simulink model "experiment_toplevel"  (R2016a)
settings: Solver=ode15s  StartTime=0.0  StopTime=20  MaxStep=1e-2  RelTol=1e-4
PreLoadFcn:
  | minitaurParameters
values from neighbouring files (symbols this model uses):
  angular_ctrl_d = 1    [minitaurParameters.m]
  angular_ctrl_i = 1    [minitaurParameters.m]
  angular_ctrl_p = 100    [minitaurParameters.m]
  enc_zero_IA = -1.25*pi    (= -3.92699081699)    [minitaurParameters.m]
  enc_zero_IB = -0.25*pi    (= -0.785398163397)    [minitaurParameters.m]
  enc_zero_IIA = 1.25*pi    (= 3.92699081699)    [minitaurParameters.m]
  enc_zero_IIB = 1.25*pi    (= 3.92699081699)    [minitaurParameters.m]
  enc_zero_IIIA = 0.5*pi    (= 1.57079632679)    [minitaurParameters.m]
  enc_zero_IIIB = 1.5*pi    (= 4.71238898038)    [minitaurParameters.m]
  enc_zero_IVA = -0.25*pi    (= -0.785398163397)    [minitaurParameters.m]
  enc_zero_IVB = 0.5*pi    (= 1.57079632679)    [minitaurParameters.m]
  fore_lag = fore_lag_vals(j)    [experiment1.m]    (also in experiment1_parfor_accelerator.m = 0; minitaurParameters.m = 0.45)
  ground_frame_depth = 0.5    [minitaurParameters.m]
  ground_length = 100    [minitaurParameters.m]
  ground_width = 10    [minitaurParameters.m]
  init_theta_IA = -pi/4    (= -0.785398163397)    [minitaurParameters.m]
  init_theta_IB = pi/4    (= 0.785398163397)    [minitaurParameters.m]
  init_theta_IIA = -pi/4    (= -0.785398163397)    [minitaurParameters.m]
  init_theta_IIB = pi/4    (= 0.785398163397)    [minitaurParameters.m]
  init_theta_IIIA = -pi/4    (= -0.785398163397)    [minitaurParameters.m]
  init_theta_IIIB = pi/4    (= 0.785398163397)    [minitaurParameters.m]
  init_theta_IVA = -pi/4    (= -0.785398163397)    [minitaurParameters.m]
  init_theta_IVB = pi/4    (= 0.785398163397)    [minitaurParameters.m]
  l1 = 100e-3    (= 0.1)    [minitaurParameters.m]
  l2 = 200e-3    (= 0.2)    [minitaurParameters.m]
  leg_joint_radius = 3e-3    (= 0.003)    [minitaurParameters.m]
  lr_sync = 1    [experiment1.m]    (also in experiment1_parfor_accelerator.m; minitaurParameters.m = 0)
  model = 'experiment_toplevel'    [experiment1_parfor_accelerator.m]
  period = period_vals(i)    [experiment1.m]    (also in experiment1_parfor_accelerator.m = 1.5; minitaurParameters.m = 0.33)
  phi_0 = 0.5*asin(l1/l2)    [experiment1.m]    (also in experiment1_parfor_accelerator.m; minitaurParameters.m)
  r_0 = l2    [experiment1.m]    (also in experiment1_parfor_accelerator.m; minitaurParameters.m = 0.2)
  r_x = 0.3*l1    [experiment1.m]    (also in experiment1_parfor_accelerator.m = 0.5*l1; minitaurParameters.m = 0.05)
  r_y = 0.2*l1    [experiment1.m]    (also in experiment1_parfor_accelerator.m = 0.3*l1; minitaurParameters.m = 0.03)
  radial_ctrl_d = 1    [minitaurParameters.m]
  radial_ctrl_i = 1    [minitaurParameters.m]
  radial_ctrl_p = 80    [minitaurParameters.m]
  safety_limit = 10e-3    (= 0.01)    [minitaurParameters.m]
undefined symbols (not defined in the file or in its folder): Axis, Fn, minitaurParams, r_stance, r_swing, stance_frac, X, Y, Z
undefined symbols (not defined in the file): leg_joint_fric_bw, leg_joint_mu_k, leg_joint_mu_s, leg_joint_vel_thresh, motor_kt, motor_kv, motor_r, motor_torque_sat
libraries: sm_lib x453, fl_lib x132, nesl_utility x31, Contact_Forces_Lib x28, simulink x19
(part 11 of 13)

== system experiment_toplevel/GR Minitaur/minitaur_leg_linkages_I/Joint Friction Model/Full ==
  Ideal Force Sensor : fl_lib/Mechanical/Mechanical Sensors/Ideal Force Sensor
  Ideal Translational Velocity Source : fl_lib/Mechanical/Mechanical Sources/Ideal Translational Velocity Source
  Joint Diameter : fl_lib/Physical Signals/Functions/PS Gain  gain=2*leg_joint_radius
  Joint Radius : fl_lib/Physical Signals/Functions/PS Gain  gain=leg_joint_radius
  Mechanical Translational Reference : fl_lib/Mechanical/Translational Elements/Mechanical Translational Reference
  Mechanical Translational Reference1 : fl_lib/Mechanical/Translational Elements/Mechanical Translational Reference
  PS Terminator : fl_lib/Physical Signals/Sinks/PS Terminator
  Translational Friction : fl_lib/Mechanical/Translational Elements/Translational Friction  brkwy_frc=mu_brk*Fn N  Col_frc=mu_k*Fn N  visc_coef=fric_visc_coeff N/(m/s)  trans_coef=trans_coeff s/m  vel_thr=linear_region_thresh m/s  v_specify=off  v_priority=None  v=0 m/s  f_specify=off  f_priority=None  f=0 N
  Joint Angular Velocity : PMIOPort  Port=1  Side=Left
  Joint Force : PMIOPort  Port=2  Side=Left
  Friction Torque : PMIOPort  Port=3  Side=Right
  connections:
  Mechanical Translational Reference/LConn1 -- Ideal Force Sensor/RConn1
  Translational Friction/LConn1 -- Ideal Force Sensor/LConn1
  Translational Friction/RConn1 -- Ideal Translational Velocity Source/LConn1
  Ideal Force Sensor/RConn2 -- Joint Diameter/LConn1
  Joint Diameter/RConn1 -- Friction Torque/RConn1
  Mechanical Translational Reference1/LConn1 -- Ideal Translational Velocity Source/RConn2
  Joint Force/RConn1 -- PS Terminator/LConn1
  Joint Radius/LConn1 -- Joint Angular Velocity/RConn1
  Joint Radius/RConn1 -- Ideal Translational Velocity Source/RConn1

== system experiment_toplevel/GR Minitaur/minitaur_leg_linkages_I/Joint Friction Model/Stick-Slip ==
  Joint Diameter : fl_lib/Physical Signals/Functions/PS Gain  gain=2*leg_joint_radius
  Joint Radius : fl_lib/Physical Signals/Functions/PS Gain  gain=leg_joint_radius
  PS Add : fl_lib/Physical Signals/Functions/PS Add
  Stick-Slip Friction X : Contact_Forces_Lib/Friction Utilities/Stick-Slip Friction 1D  fn_axis=X-Axis  mu_kinetic=mu_k/2  mu_static=mu_s/2  vel_th=linear_region_thresh  filt_const=1/(2*pi*fric_bandwidth)
  Stick-Slip Friction Y : Contact_Forces_Lib/Friction Utilities/Stick-Slip Friction 1D  fn_axis=Y-Axis  mu_kinetic=mu_k/2  mu_static=mu_s/2  vel_th=linear_region_thresh  filt_const=1/(2*pi*fric_bandwidth)
  Joint Angular Velocity : PMIOPort  Port=1  Side=Left
  Joint Force : PMIOPort  Port=2  Side=Left
  Friction Torque : PMIOPort  Port=3  Side=Right
  connections:
  Stick-Slip Friction X/LConn2 -- Stick-Slip Friction Y/LConn2 -- Joint Radius/RConn1
  Joint Force/RConn1 -- Stick-Slip Friction Y/LConn1 -- Stick-Slip Friction X/LConn1
  Stick-Slip Friction Y/RConn1 -- PS Add/LConn2
  Stick-Slip Friction X/RConn1 -- PS Add/LConn1
  Joint Diameter/LConn1 -- PS Add/RConn1
  Joint Diameter/RConn1 -- Friction Torque/RConn1
  Joint Radius/LConn1 -- Joint Angular Velocity/RConn1

== system experiment_toplevel/GR Minitaur/minitaur_leg_linkages_I/Joint Friction Model1/Full ==
  Ideal Force Sensor : fl_lib/Mechanical/Mechanical Sensors/Ideal Force Sensor
  Ideal Translational Velocity Source : fl_lib/Mechanical/Mechanical Sources/Ideal Translational Velocity Source
  Joint Diameter : fl_lib/Physical Signals/Functions/PS Gain  gain=2*leg_joint_radius
  Joint Radius : fl_lib/Physical Signals/Functions/PS Gain  gain=leg_joint_radius
  Mechanical Translational Reference : fl_lib/Mechanical/Translational Elements/Mechanical Translational Reference
  Mechanical Translational Reference1 : fl_lib/Mechanical/Translational Elements/Mechanical Translational Reference
  PS Terminator : fl_lib/Physical Signals/Sinks/PS Terminator
  Translational Friction : fl_lib/Mechanical/Translational Elements/Translational Friction  brkwy_frc=mu_brk*Fn N  Col_frc=mu_k*Fn N  visc_coef=fric_visc_coeff N/(m/s)  trans_coef=trans_coeff s/m  vel_thr=linear_region_thresh m/s  v_specify=off  v_priority=None  v=0 m/s  f_specify=off  f_priority=None  f=0 N
  Joint Angular Velocity : PMIOPort  Port=1  Side=Left
  Joint Force : PMIOPort  Port=2  Side=Left
  Friction Torque : PMIOPort  Port=3  Side=Right
  connections:
  Mechanical Translational Reference/LConn1 -- Ideal Force Sensor/RConn1
  Translational Friction/LConn1 -- Ideal Force Sensor/LConn1
  Translational Friction/RConn1 -- Ideal Translational Velocity Source/LConn1
  Ideal Force Sensor/RConn2 -- Joint Diameter/LConn1
  Joint Diameter/RConn1 -- Friction Torque/RConn1
  Mechanical Translational Reference1/LConn1 -- Ideal Translational Velocity Source/RConn2
  Joint Force/RConn1 -- PS Terminator/LConn1
  Joint Radius/LConn1 -- Joint Angular Velocity/RConn1
  Joint Radius/RConn1 -- Ideal Translational Velocity Source/RConn1

== system experiment_toplevel/GR Minitaur/minitaur_leg_linkages_I/Joint Friction Model1/Stick-Slip ==
  Joint Diameter : fl_lib/Physical Signals/Functions/PS Gain  gain=2*leg_joint_radius
  Joint Radius : fl_lib/Physical Signals/Functions/PS Gain  gain=leg_joint_radius
  PS Add : fl_lib/Physical Signals/Functions/PS Add
  Stick-Slip Friction X : Contact_Forces_Lib/Friction Utilities/Stick-Slip Friction 1D  fn_axis=X-Axis  mu_kinetic=mu_k/2  mu_static=mu_s/2  vel_th=linear_region_thresh  filt_const=1/(2*pi*fric_bandwidth)
  Stick-Slip Friction Y : Contact_Forces_Lib/Friction Utilities/Stick-Slip Friction 1D  fn_axis=Y-Axis  mu_kinetic=mu_k/2  mu_static=mu_s/2  vel_th=linear_region_thresh  filt_const=1/(2*pi*fric_bandwidth)
  Joint Angular Velocity : PMIOPort  Port=1  Side=Left
  Joint Force : PMIOPort  Port=2  Side=Left
  Friction Torque : PMIOPort  Port=3  Side=Right
  connections:
  Joint Radius/RConn1 -- Stick-Slip Friction X/LConn2 -- Stick-Slip Friction Y/LConn2
  Joint Force/RConn1 -- Stick-Slip Friction X/LConn1 -- Stick-Slip Friction Y/LConn1
  Stick-Slip Friction Y/RConn1 -- PS Add/LConn2
  Stick-Slip Friction X/RConn1 -- PS Add/LConn1
  Joint Diameter/LConn1 -- PS Add/RConn1
  Joint Diameter/RConn1 -- Friction Torque/RConn1
  Joint Radius/LConn1 -- Joint Angular Velocity/RConn1

== system experiment_toplevel/GR Minitaur/minitaur_leg_linkages_I/Joint Friction Model2/Full ==
  Ideal Force Sensor : fl_lib/Mechanical/Mechanical Sensors/Ideal Force Sensor
  Ideal Translational Velocity Source : fl_lib/Mechanical/Mechanical Sources/Ideal Translational Velocity Source
  Joint Diameter : fl_lib/Physical Signals/Functions/PS Gain  gain=2*leg_joint_radius
  Joint Radius : fl_lib/Physical Signals/Functions/PS Gain  gain=leg_joint_radius
  Mechanical Translational Reference : fl_lib/Mechanical/Translational Elements/Mechanical Translational Reference
  Mechanical Translational Reference1 : fl_lib/Mechanical/Translational Elements/Mechanical Translational Reference
  PS Terminator : fl_lib/Physical Signals/Sinks/PS Terminator
  Translational Friction : fl_lib/Mechanical/Translational Elements/Translational Friction  brkwy_frc=mu_brk*Fn N  Col_frc=mu_k*Fn N  visc_coef=fric_visc_coeff N/(m/s)  trans_coef=trans_coeff s/m  vel_thr=linear_region_thresh m/s  v_specify=off  v_priority=None  v=0 m/s  f_specify=off  f_priority=None  f=0 N
  Joint Angular Velocity : PMIOPort  Port=1  Side=Left
  Joint Force : PMIOPort  Port=2  Side=Left
  Friction Torque : PMIOPort  Port=3  Side=Right
  connections:
  Mechanical Translational Reference/LConn1 -- Ideal Force Sensor/RConn1
  Translational Friction/LConn1 -- Ideal Force Sensor/LConn1
  Translational Friction/RConn1 -- Ideal Translational Velocity Source/LConn1
  Ideal Force Sensor/RConn2 -- Joint Diameter/LConn1
  Joint Diameter/RConn1 -- Friction Torque/RConn1
  Mechanical Translational Reference1/LConn1 -- Ideal Translational Velocity Source/RConn2
  Joint Force/RConn1 -- PS Terminator/LConn1
  Joint Radius/LConn1 -- Joint Angular Velocity/RConn1
  Joint Radius/RConn1 -- Ideal Translational Velocity Source/RConn1

== system experiment_toplevel/GR Minitaur/minitaur_leg_linkages_I/Joint Friction Model2/Stick-Slip ==
  Joint Diameter : fl_lib/Physical Signals/Functions/PS Gain  gain=2*leg_joint_radius
  Joint Radius : fl_lib/Physical Signals/Functions/PS Gain  gain=leg_joint_radius
  PS Add : fl_lib/Physical Signals/Functions/PS Add
  Stick-Slip Friction X : Contact_Forces_Lib/Friction Utilities/Stick-Slip Friction 1D  fn_axis=X-Axis  mu_kinetic=mu_k/2  mu_static=mu_s/2  vel_th=linear_region_thresh  filt_const=1/(2*pi*fric_bandwidth)
  Stick-Slip Friction Y : Contact_Forces_Lib/Friction Utilities/Stick-Slip Friction 1D  fn_axis=Y-Axis  mu_kinetic=mu_k/2  mu_static=mu_s/2  vel_th=linear_region_thresh  filt_const=1/(2*pi*fric_bandwidth)
  Joint Angular Velocity : PMIOPort  Port=1  Side=Left
  Joint Force : PMIOPort  Port=2  Side=Left
  Friction Torque : PMIOPort  Port=3  Side=Right
  connections:
  Joint Radius/RConn1 -- Stick-Slip Friction X/LConn2 -- Stick-Slip Friction Y/LConn2
  Joint Force/RConn1 -- Stick-Slip Friction X/LConn1 -- Stick-Slip Friction Y/LConn1
  Stick-Slip Friction Y/RConn1 -- PS Add/LConn2
  Stick-Slip Friction X/RConn1 -- PS Add/LConn1
  Joint Diameter/LConn1 -- PS Add/RConn1
  Joint Diameter/RConn1 -- Friction Torque/RConn1
  Joint Radius/LConn1 -- Joint Angular Velocity/RConn1

== system experiment_toplevel/GR Minitaur/minitaur_leg_linkages_II/Joint Friction Model/Full ==
  Ideal Force Sensor : fl_lib/Mechanical/Mechanical Sensors/Ideal Force Sensor
  Ideal Translational Velocity Source : fl_lib/Mechanical/Mechanical Sources/Ideal Translational Velocity Source
  Joint Diameter : fl_lib/Physical Signals/Functions/PS Gain  gain=2*leg_joint_radius
  Joint Radius : fl_lib/Physical Signals/Functions/PS Gain  gain=leg_joint_radius
  Mechanical Translational Reference : fl_lib/Mechanical/Translational Elements/Mechanical Translational Reference
  Mechanical Translational Reference1 : fl_lib/Mechanical/Translational Elements/Mechanical Translational Reference
  PS Terminator : fl_lib/Physical Signals/Sinks/PS Terminator
  Translational Friction : fl_lib/Mechanical/Translational Elements/Translational Friction  brkwy_frc=mu_brk*Fn N  Col_frc=mu_k*Fn N  visc_coef=fric_visc_coeff N/(m/s)  trans_coef=trans_coeff s/m  vel_thr=linear_region_thresh m/s  v_specify=off  v_priority=None  v=0 m/s  f_specify=off  f_priority=None  f=0 N
  Joint Angular Velocity : PMIOPort  Port=1  Side=Left
  Joint Force : PMIOPort  Port=2  Side=Left
  Friction Torque : PMIOPort  Port=3  Side=Right
  connections:
  Mechanical Translational Reference/LConn1 -- Ideal Force Sensor/RConn1
  Translational Friction/LConn1 -- Ideal Force Sensor/LConn1
  Translational Friction/RConn1 -- Ideal Translational Velocity Source/LConn1
  Ideal Force Sensor/RConn2 -- Joint Diameter/LConn1
  Joint Diameter/RConn1 -- Friction Torque/RConn1
  Mechanical Translational Reference1/LConn1 -- Ideal Translational Velocity Source/RConn2
  Joint Force/RConn1 -- PS Terminator/LConn1
  Joint Radius/LConn1 -- Joint Angular Velocity/RConn1
  Joint Radius/RConn1 -- Ideal Translational Velocity Source/RConn1

== system experiment_toplevel/GR Minitaur/minitaur_leg_linkages_II/Joint Friction Model/Stick-Slip ==
  Joint Diameter : fl_lib/Physical Signals/Functions/PS Gain  gain=2*leg_joint_radius
  Joint Radius : fl_lib/Physical Signals/Functions/PS Gain  gain=leg_joint_radius
  PS Add : fl_lib/Physical Signals/Functions/PS Add
  Stick-Slip Friction X : Contact_Forces_Lib/Friction Utilities/Stick-Slip Friction 1D  fn_axis=X-Axis  mu_kinetic=mu_k/2  mu_static=mu_s/2  vel_th=linear_region_thresh  filt_const=1/(2*pi*fric_bandwidth)
  Stick-Slip Friction Y : Contact_Forces_Lib/Friction Utilities/Stick-Slip Friction 1D  fn_axis=Y-Axis  mu_kinetic=mu_k/2  mu_static=mu_s/2  vel_th=linear_region_thresh  filt_const=1/(2*pi*fric_bandwidth)
  Joint Angular Velocity : PMIOPort  Port=1  Side=Left
  Joint Force : PMIOPort  Port=2  Side=Left
  Friction Torque : PMIOPort  Port=3  Side=Right
  connections:
  Joint Radius/RConn1 -- Stick-Slip Friction X/LConn2 -- Stick-Slip Friction Y/LConn2
  Joint Force/RConn1 -- Stick-Slip Friction X/LConn1 -- Stick-Slip Friction Y/LConn1
  Stick-Slip Friction Y/RConn1 -- PS Add/LConn2
  Stick-Slip Friction X/RConn1 -- PS Add/LConn1
  Joint Diameter/LConn1 -- PS Add/RConn1
  Joint Diameter/RConn1 -- Friction Torque/RConn1
  Joint Radius/LConn1 -- Joint Angular Velocity/RConn1

== system experiment_toplevel/GR Minitaur/minitaur_leg_linkages_II/Joint Friction Model1/Full ==
  Ideal Force Sensor : fl_lib/Mechanical/Mechanical Sensors/Ideal Force Sensor
  Ideal Translational Velocity Source : fl_lib/Mechanical/Mechanical Sources/Ideal Translational Velocity Source
  Joint Diameter : fl_lib/Physical Signals/Functions/PS Gain  gain=2*leg_joint_radius
  Joint Radius : fl_lib/Physical Signals/Functions/PS Gain  gain=leg_joint_radius
  Mechanical Translational Reference : fl_lib/Mechanical/Translational Elements/Mechanical Translational Reference
  Mechanical Translational Reference1 : fl_lib/Mechanical/Translational Elements/Mechanical Translational Reference
  PS Terminator : fl_lib/Physical Signals/Sinks/PS Terminator
  Translational Friction : fl_lib/Mechanical/Translational Elements/Translational Friction  brkwy_frc=mu_brk*Fn N  Col_frc=mu_k*Fn N  visc_coef=fric_visc_coeff N/(m/s)  trans_coef=trans_coeff s/m  vel_thr=linear_region_thresh m/s  v_specify=off  v_priority=None  v=0 m/s  f_specify=off  f_priority=None  f=0 N
  Joint Angular Velocity : PMIOPort  Port=1  Side=Left
  Joint Force : PMIOPort  Port=2  Side=Left
  Friction Torque : PMIOPort  Port=3  Side=Right
  connections:
  Mechanical Translational Reference/LConn1 -- Ideal Force Sensor/RConn1
  Translational Friction/LConn1 -- Ideal Force Sensor/LConn1
  Translational Friction/RConn1 -- Ideal Translational Velocity Source/LConn1
  Ideal Force Sensor/RConn2 -- Joint Diameter/LConn1
  Joint Diameter/RConn1 -- Friction Torque/RConn1
  Mechanical Translational Reference1/LConn1 -- Ideal Translational Velocity Source/RConn2
  Joint Force/RConn1 -- PS Terminator/LConn1
  Joint Radius/LConn1 -- Joint Angular Velocity/RConn1
  Joint Radius/RConn1 -- Ideal Translational Velocity Source/RConn1

== system experiment_toplevel/GR Minitaur/minitaur_leg_linkages_II/Joint Friction Model1/Stick-Slip ==
  Joint Diameter : fl_lib/Physical Signals/Functions/PS Gain  gain=2*leg_joint_radius
  Joint Radius : fl_lib/Physical Signals/Functions/PS Gain  gain=leg_joint_radius
  PS Add : fl_lib/Physical Signals/Functions/PS Add
  Stick-Slip Friction X : Contact_Forces_Lib/Friction Utilities/Stick-Slip Friction 1D  fn_axis=X-Axis  mu_kinetic=mu_k/2  mu_static=mu_s/2  vel_th=linear_region_thresh  filt_const=1/(2*pi*fric_bandwidth)
  Stick-Slip Friction Y : Contact_Forces_Lib/Friction Utilities/Stick-Slip Friction 1D  fn_axis=Y-Axis  mu_kinetic=mu_k/2  mu_static=mu_s/2  vel_th=linear_region_thresh  filt_const=1/(2*pi*fric_bandwidth)
  Joint Angular Velocity : PMIOPort  Port=1  Side=Left
  Joint Force : PMIOPort  Port=2  Side=Left
  Friction Torque : PMIOPort  Port=3  Side=Right
  connections:
  Joint Radius/RConn1 -- Stick-Slip Friction X/LConn2 -- Stick-Slip Friction Y/LConn2
  Joint Force/RConn1 -- Stick-Slip Friction X/LConn1 -- Stick-Slip Friction Y/LConn1
  Stick-Slip Friction Y/RConn1 -- PS Add/LConn2
  Stick-Slip Friction X/RConn1 -- PS Add/LConn1
  Joint Diameter/LConn1 -- PS Add/RConn1
  Joint Diameter/RConn1 -- Friction Torque/RConn1
  Joint Radius/LConn1 -- Joint Angular Velocity/RConn1

== system experiment_toplevel/GR Minitaur/minitaur_leg_linkages_II/Joint Friction Model2/Full ==
  Ideal Force Sensor : fl_lib/Mechanical/Mechanical Sensors/Ideal Force Sensor
  Ideal Translational Velocity Source : fl_lib/Mechanical/Mechanical Sources/Ideal Translational Velocity Source
  Joint Diameter : fl_lib/Physical Signals/Functions/PS Gain  gain=2*leg_joint_radius
  Joint Radius : fl_lib/Physical Signals/Functions/PS Gain  gain=leg_joint_radius
  Mechanical Translational Reference : fl_lib/Mechanical/Translational Elements/Mechanical Translational Reference
  Mechanical Translational Reference1 : fl_lib/Mechanical/Translational Elements/Mechanical Translational Reference
  PS Terminator : fl_lib/Physical Signals/Sinks/PS Terminator
  Translational Friction : fl_lib/Mechanical/Translational Elements/Translational Friction  brkwy_frc=mu_brk*Fn N  Col_frc=mu_k*Fn N  visc_coef=fric_visc_coeff N/(m/s)  trans_coef=trans_coeff s/m  vel_thr=linear_region_thresh m/s  v_specify=off  v_priority=None  v=0 m/s  f_specify=off  f_priority=None  f=0 N
  Joint Angular Velocity : PMIOPort  Port=1  Side=Left
  Joint Force : PMIOPort  Port=2  Side=Left
  Friction Torque : PMIOPort  Port=3  Side=Right
  connections:
  Mechanical Translational Reference/LConn1 -- Ideal Force Sensor/RConn1
  Translational Friction/LConn1 -- Ideal Force Sensor/LConn1
  Translational Friction/RConn1 -- Ideal Translational Velocity Source/LConn1
  Ideal Force Sensor/RConn2 -- Joint Diameter/LConn1
  Joint Diameter/RConn1 -- Friction Torque/RConn1
  Mechanical Translational Reference1/LConn1 -- Ideal Translational Velocity Source/RConn2
  Joint Force/RConn1 -- PS Terminator/LConn1
  Joint Radius/LConn1 -- Joint Angular Velocity/RConn1
  Joint Radius/RConn1 -- Ideal Translational Velocity Source/RConn1

== system experiment_toplevel/GR Minitaur/minitaur_leg_linkages_II/Joint Friction Model2/Stick-Slip ==
  Joint Diameter : fl_lib/Physical Signals/Functions/PS Gain  gain=2*leg_joint_radius
  Joint Radius : fl_lib/Physical Signals/Functions/PS Gain  gain=leg_joint_radius
  PS Add : fl_lib/Physical Signals/Functions/PS Add
  Stick-Slip Friction X : Contact_Forces_Lib/Friction Utilities/Stick-Slip Friction 1D  fn_axis=X-Axis  mu_kinetic=mu_k/2  mu_static=mu_s/2  vel_th=linear_region_thresh  filt_const=1/(2*pi*fric_bandwidth)
  Stick-Slip Friction Y : Contact_Forces_Lib/Friction Utilities/Stick-Slip Friction 1D  fn_axis=Y-Axis  mu_kinetic=mu_k/2  mu_static=mu_s/2  vel_th=linear_region_thresh  filt_const=1/(2*pi*fric_bandwidth)
  Joint Angular Velocity : PMIOPort  Port=1  Side=Left
  Joint Force : PMIOPort  Port=2  Side=Left
  Friction Torque : PMIOPort  Port=3  Side=Right
  connections:
  Joint Radius/RConn1 -- Stick-Slip Friction X/LConn2 -- Stick-Slip Friction Y/LConn2
  Joint Force/RConn1 -- Stick-Slip Friction X/LConn1 -- Stick-Slip Friction Y/LConn1
  Stick-Slip Friction Y/RConn1 -- PS Add/LConn2
  Stick-Slip Friction X/RConn1 -- PS Add/LConn1
  Joint Diameter/LConn1 -- PS Add/RConn1
  Joint Diameter/RConn1 -- Friction Torque/RConn1
  Joint Radius/LConn1 -- Joint Angular Velocity/RConn1

== system experiment_toplevel/GR Minitaur/minitaur_leg_linkages_III/Joint Friction Model/Full ==
  Ideal Force Sensor : fl_lib/Mechanical/Mechanical Sensors/Ideal Force Sensor
  Ideal Translational Velocity Source : fl_lib/Mechanical/Mechanical Sources/Ideal Translational Velocity Source
  Joint Diameter : fl_lib/Physical Signals/Functions/PS Gain  gain=2*leg_joint_radius
  Joint Radius : fl_lib/Physical Signals/Functions/PS Gain  gain=leg_joint_radius
  Mechanical Translational Reference : fl_lib/Mechanical/Translational Elements/Mechanical Translational Reference
  Mechanical Translational Reference1 : fl_lib/Mechanical/Translational Elements/Mechanical Translational Reference
  PS Terminator : fl_lib/Physical Signals/Sinks/PS Terminator
  Translational Friction : fl_lib/Mechanical/Translational Elements/Translational Friction  brkwy_frc=mu_brk*Fn N  Col_frc=mu_k*Fn N  visc_coef=fric_visc_coeff N/(m/s)  trans_coef=trans_coeff s/m  vel_thr=linear_region_thresh m/s  v_specify=off  v_priority=None  v=0 m/s  f_specify=off  f_priority=None  f=0 N
  Joint Angular Velocity : PMIOPort  Port=1  Side=Left
  Joint Force : PMIOPort  Port=2  Side=Left
  Friction Torque : PMIOPort  Port=3  Side=Right
  connections:
  Mechanical Translational Reference/LConn1 -- Ideal Force Sensor/RConn1
  Translational Friction/LConn1 -- Ideal Force Sensor/LConn1
  Translational Friction/RConn1 -- Ideal Translational Velocity Source/LConn1
  Ideal Force Sensor/RConn2 -- Joint Diameter/LConn1
  Joint Diameter/RConn1 -- Friction Torque/RConn1
  Mechanical Translational Reference1/LConn1 -- Ideal Translational Velocity Source/RConn2
  Joint Force/RConn1 -- PS Terminator/LConn1
  Joint Radius/LConn1 -- Joint Angular Velocity/RConn1
  Joint Radius/RConn1 -- Ideal Translational Velocity Source/RConn1

== system experiment_toplevel/GR Minitaur/minitaur_leg_linkages_III/Joint Friction Model/Stick-Slip ==
  Joint Diameter : fl_lib/Physical Signals/Functions/PS Gain  gain=2*leg_joint_radius
  Joint Radius : fl_lib/Physical Signals/Functions/PS Gain  gain=leg_joint_radius
  PS Add : fl_lib/Physical Signals/Functions/PS Add
  Stick-Slip Friction X : Contact_Forces_Lib/Friction Utilities/Stick-Slip Friction 1D  fn_axis=X-Axis  mu_kinetic=mu_k/2  mu_static=mu_s/2  vel_th=linear_region_thresh  filt_const=1/(2*pi*fric_bandwidth)
  Stick-Slip Friction Y : Contact_Forces_Lib/Friction Utilities/Stick-Slip Friction 1D  fn_axis=Y-Axis  mu_kinetic=mu_k/2  mu_static=mu_s/2  vel_th=linear_region_thresh  filt_const=1/(2*pi*fric_bandwidth)
  Joint Angular Velocity : PMIOPort  Port=1  Side=Left
  Joint Force : PMIOPort  Port=2  Side=Left
  Friction Torque : PMIOPort  Port=3  Side=Right
  connections:
  Joint Radius/RConn1 -- Stick-Slip Friction X/LConn2 -- Stick-Slip Friction Y/LConn2
  Joint Force/RConn1 -- Stick-Slip Friction X/LConn1 -- Stick-Slip Friction Y/LConn1
  Stick-Slip Friction Y/RConn1 -- PS Add/LConn2
  Stick-Slip Friction X/RConn1 -- PS Add/LConn1
  Joint Diameter/LConn1 -- PS Add/RConn1
  Joint Diameter/RConn1 -- Friction Torque/RConn1
  Joint Radius/LConn1 -- Joint Angular Velocity/RConn1

== system experiment_toplevel/GR Minitaur/minitaur_leg_linkages_III/Joint Friction Model1/Full ==
  Ideal Force Sensor : fl_lib/Mechanical/Mechanical Sensors/Ideal Force Sensor
  Ideal Translational Velocity Source : fl_lib/Mechanical/Mechanical Sources/Ideal Translational Velocity Source
  Joint Diameter : fl_lib/Physical Signals/Functions/PS Gain  gain=2*leg_joint_radius
  Joint Radius : fl_lib/Physical Signals/Functions/PS Gain  gain=leg_joint_radius
  Mechanical Translational Reference : fl_lib/Mechanical/Translational Elements/Mechanical Translational Reference
  Mechanical Translational Reference1 : fl_lib/Mechanical/Translational Elements/Mechanical Translational Reference
  PS Terminator : fl_lib/Physical Signals/Sinks/PS Terminator
  Translational Friction : fl_lib/Mechanical/Translational Elements/Translational Friction  brkwy_frc=mu_brk*Fn N  Col_frc=mu_k*Fn N  visc_coef=fric_visc_coeff N/(m/s)  trans_coef=trans_coeff s/m  vel_thr=linear_region_thresh m/s  v_specify=off  v_priority=None  v=0 m/s  f_specify=off  f_priority=None  f=0 N
  Joint Angular Velocity : PMIOPort  Port=1  Side=Left
  Joint Force : PMIOPort  Port=2  Side=Left
  Friction Torque : PMIOPort  Port=3  Side=Right
  connections:
  Mechanical Translational Reference/LConn1 -- Ideal Force Sensor/RConn1
  Translational Friction/LConn1 -- Ideal Force Sensor/LConn1
  Translational Friction/RConn1 -- Ideal Translational Velocity Source/LConn1
  Ideal Force Sensor/RConn2 -- Joint Diameter/LConn1
  Joint Diameter/RConn1 -- Friction Torque/RConn1
  Mechanical Translational Reference1/LConn1 -- Ideal Translational Velocity Source/RConn2
  Joint Force/RConn1 -- PS Terminator/LConn1
  Joint Radius/LConn1 -- Joint Angular Velocity/RConn1
  Joint Radius/RConn1 -- Ideal Translational Velocity Source/RConn1

== system experiment_toplevel/GR Minitaur/minitaur_leg_linkages_III/Joint Friction Model1/Stick-Slip ==
  Joint Diameter : fl_lib/Physical Signals/Functions/PS Gain  gain=2*leg_joint_radius
  Joint Radius : fl_lib/Physical Signals/Functions/PS Gain  gain=leg_joint_radius
  PS Add : fl_lib/Physical Signals/Functions/PS Add
  Stick-Slip Friction X : Contact_Forces_Lib/Friction Utilities/Stick-Slip Friction 1D  fn_axis=X-Axis  mu_kinetic=mu_k/2  mu_static=mu_s/2  vel_th=linear_region_thresh  filt_const=1/(2*pi*fric_bandwidth)
  Stick-Slip Friction Y : Contact_Forces_Lib/Friction Utilities/Stick-Slip Friction 1D  fn_axis=Y-Axis  mu_kinetic=mu_k/2  mu_static=mu_s/2  vel_th=linear_region_thresh  filt_const=1/(2*pi*fric_bandwidth)
  Joint Angular Velocity : PMIOPort  Port=1  Side=Left
  Joint Force : PMIOPort  Port=2  Side=Left
  Friction Torque : PMIOPort  Port=3  Side=Right
  connections:
  Joint Radius/RConn1 -- Stick-Slip Friction X/LConn2 -- Stick-Slip Friction Y/LConn2
  Joint Force/RConn1 -- Stick-Slip Friction X/LConn1 -- Stick-Slip Friction Y/LConn1
  Stick-Slip Friction Y/RConn1 -- PS Add/LConn2
  Stick-Slip Friction X/RConn1 -- PS Add/LConn1
  Joint Diameter/LConn1 -- PS Add/RConn1
  Joint Diameter/RConn1 -- Friction Torque/RConn1
  Joint Radius/LConn1 -- Joint Angular Velocity/RConn1

== system experiment_toplevel/GR Minitaur/minitaur_leg_linkages_III/Joint Friction Model2/Full ==
  Ideal Force Sensor : fl_lib/Mechanical/Mechanical Sensors/Ideal Force Sensor
  Ideal Translational Velocity Source : fl_lib/Mechanical/Mechanical Sources/Ideal Translational Velocity Source
  Joint Diameter : fl_lib/Physical Signals/Functions/PS Gain  gain=2*leg_joint_radius
  Joint Radius : fl_lib/Physical Signals/Functions/PS Gain  gain=leg_joint_radius
  Mechanical Translational Reference : fl_lib/Mechanical/Translational Elements/Mechanical Translational Reference
  Mechanical Translational Reference1 : fl_lib/Mechanical/Translational Elements/Mechanical Translational Reference
  PS Terminator : fl_lib/Physical Signals/Sinks/PS Terminator
  Translational Friction : fl_lib/Mechanical/Translational Elements/Translational Friction  brkwy_frc=mu_brk*Fn N  Col_frc=mu_k*Fn N  visc_coef=fric_visc_coeff N/(m/s)  trans_coef=trans_coeff s/m  vel_thr=linear_region_thresh m/s  v_specify=off  v_priority=None  v=0 m/s  f_specify=off  f_priority=None  f=0 N
  Joint Angular Velocity : PMIOPort  Port=1  Side=Left
  Joint Force : PMIOPort  Port=2  Side=Left
  Friction Torque : PMIOPort  Port=3  Side=Right
  connections:
  Mechanical Translational Reference/LConn1 -- Ideal Force Sensor/RConn1
  Translational Friction/LConn1 -- Ideal Force Sensor/LConn1
  Translational Friction/RConn1 -- Ideal Translational Velocity Source/LConn1
  Ideal Force Sensor/RConn2 -- Joint Diameter/LConn1
  Joint Diameter/RConn1 -- Friction Torque/RConn1
  Mechanical Translational Reference1/LConn1 -- Ideal Translational Velocity Source/RConn2
  Joint Force/RConn1 -- PS Terminator/LConn1
  Joint Radius/LConn1 -- Joint Angular Velocity/RConn1
  Joint Radius/RConn1 -- Ideal Translational Velocity Source/RConn1

== system experiment_toplevel/GR Minitaur/minitaur_leg_linkages_III/Joint Friction Model2/Stick-Slip ==
  Joint Diameter : fl_lib/Physical Signals/Functions/PS Gain  gain=2*leg_joint_radius
  Joint Radius : fl_lib/Physical Signals/Functions/PS Gain  gain=leg_joint_radius
  PS Add : fl_lib/Physical Signals/Functions/PS Add
  Stick-Slip Friction X : Contact_Forces_Lib/Friction Utilities/Stick-Slip Friction 1D  fn_axis=X-Axis  mu_kinetic=mu_k/2  mu_static=mu_s/2  vel_th=linear_region_thresh  filt_const=1/(2*pi*fric_bandwidth)
  Stick-Slip Friction Y : Contact_Forces_Lib/Friction Utilities/Stick-Slip Friction 1D  fn_axis=Y-Axis  mu_kinetic=mu_k/2  mu_static=mu_s/2  vel_th=linear_region_thresh  filt_const=1/(2*pi*fric_bandwidth)
  Joint Angular Velocity : PMIOPort  Port=1  Side=Left
  Joint Force : PMIOPort  Port=2  Side=Left
  Friction Torque : PMIOPort  Port=3  Side=Right
  connections:
  Joint Radius/RConn1 -- Stick-Slip Friction X/LConn2 -- Stick-Slip Friction Y/LConn2
  Joint Force/RConn1 -- Stick-Slip Friction X/LConn1 -- Stick-Slip Friction Y/LConn1
  Stick-Slip Friction Y/RConn1 -- PS Add/LConn2
  Stick-Slip Friction X/RConn1 -- PS Add/LConn1
  Joint Diameter/LConn1 -- PS Add/RConn1
  Joint Diameter/RConn1 -- Friction Torque/RConn1
  Joint Radius/LConn1 -- Joint Angular Velocity/RConn1

== system experiment_toplevel/GR Minitaur/minitaur_leg_linkages_IV/Joint Friction Model/Full ==
  Ideal Force Sensor : fl_lib/Mechanical/Mechanical Sensors/Ideal Force Sensor
  Ideal Translational Velocity Source : fl_lib/Mechanical/Mechanical Sources/Ideal Translational Velocity Source
  Joint Diameter : fl_lib/Physical Signals/Functions/PS Gain  gain=2*leg_joint_radius
  Joint Radius : fl_lib/Physical Signals/Functions/PS Gain  gain=leg_joint_radius
  Mechanical Translational Reference : fl_lib/Mechanical/Translational Elements/Mechanical Translational Reference
  Mechanical Translational Reference1 : fl_lib/Mechanical/Translational Elements/Mechanical Translational Reference
  PS Terminator : fl_lib/Physical Signals/Sinks/PS Terminator
  Translational Friction : fl_lib/Mechanical/Translational Elements/Translational Friction  brkwy_frc=mu_brk*Fn N  Col_frc=mu_k*Fn N  visc_coef=fric_visc_coeff N/(m/s)  trans_coef=trans_coeff s/m  vel_thr=linear_region_thresh m/s  v_specify=off  v_priority=None  v=0 m/s  f_specify=off  f_priority=None  f=0 N
  Joint Angular Velocity : PMIOPort  Port=1  Side=Left
  Joint Force : PMIOPort  Port=2  Side=Left
  Friction Torque : PMIOPort  Port=3  Side=Right
  connections:
  Mechanical Translational Reference/LConn1 -- Ideal Force Sensor/RConn1
  Translational Friction/LConn1 -- Ideal Force Sensor/LConn1
  Translational Friction/RConn1 -- Ideal Translational Velocity Source/LConn1
  Ideal Force Sensor/RConn2 -- Joint Diameter/LConn1
  Joint Diameter/RConn1 -- Friction Torque/RConn1
  Mechanical Translational Reference1/LConn1 -- Ideal Translational Velocity Source/RConn2
  Joint Force/RConn1 -- PS Terminator/LConn1
  Joint Radius/LConn1 -- Joint Angular Velocity/RConn1
  Joint Radius/RConn1 -- Ideal Translational Velocity Source/RConn1

== system experiment_toplevel/GR Minitaur/minitaur_leg_linkages_IV/Joint Friction Model/Stick-Slip ==
  Joint Diameter : fl_lib/Physical Signals/Functions/PS Gain  gain=2*leg_joint_radius
  Joint Radius : fl_lib/Physical Signals/Functions/PS Gain  gain=leg_joint_radius
  PS Add : fl_lib/Physical Signals/Functions/PS Add
  Stick-Slip Friction X : Contact_Forces_Lib/Friction Utilities/Stick-Slip Friction 1D  fn_axis=X-Axis  mu_kinetic=mu_k/2  mu_static=mu_s/2  vel_th=linear_region_thresh  filt_const=1/(2*pi*fric_bandwidth)
  Stick-Slip Friction Y : Contact_Forces_Lib/Friction Utilities/Stick-Slip Friction 1D  fn_axis=Y-Axis  mu_kinetic=mu_k/2  mu_static=mu_s/2  vel_th=linear_region_thresh  filt_const=1/(2*pi*fric_bandwidth)
  Joint Angular Velocity : PMIOPort  Port=1  Side=Left
  Joint Force : PMIOPort  Port=2  Side=Left
  Friction Torque : PMIOPort  Port=3  Side=Right
  connections:
  Joint Radius/RConn1 -- Stick-Slip Friction X/LConn2 -- Stick-Slip Friction Y/LConn2
  Joint Force/RConn1 -- Stick-Slip Friction X/LConn1 -- Stick-Slip Friction Y/LConn1
  Stick-Slip Friction Y/RConn1 -- PS Add/LConn2
  Stick-Slip Friction X/RConn1 -- PS Add/LConn1
  Joint Diameter/LConn1 -- PS Add/RConn1
  Joint Diameter/RConn1 -- Friction Torque/RConn1
  Joint Radius/LConn1 -- Joint Angular Velocity/RConn1

== system experiment_toplevel/GR Minitaur/minitaur_leg_linkages_IV/Joint Friction Model1/Full ==
  Ideal Force Sensor : fl_lib/Mechanical/Mechanical Sensors/Ideal Force Sensor
  Ideal Translational Velocity Source : fl_lib/Mechanical/Mechanical Sources/Ideal Translational Velocity Source
  Joint Diameter : fl_lib/Physical Signals/Functions/PS Gain  gain=2*leg_joint_radius
  Joint Radius : fl_lib/Physical Signals/Functions/PS Gain  gain=leg_joint_radius
  Mechanical Translational Reference : fl_lib/Mechanical/Translational Elements/Mechanical Translational Reference
  Mechanical Translational Reference1 : fl_lib/Mechanical/Translational Elements/Mechanical Translational Reference
  PS Terminator : fl_lib/Physical Signals/Sinks/PS Terminator
  Translational Friction : fl_lib/Mechanical/Translational Elements/Translational Friction  brkwy_frc=mu_brk*Fn N  Col_frc=mu_k*Fn N  visc_coef=fric_visc_coeff N/(m/s)  trans_coef=trans_coeff s/m  vel_thr=linear_region_thresh m/s  v_specify=off  v_priority=None  v=0 m/s  f_specify=off  f_priority=None  f=0 N
  Joint Angular Velocity : PMIOPort  Port=1  Side=Left
  Joint Force : PMIOPort  Port=2  Side=Left
  Friction Torque : PMIOPort  Port=3  Side=Right
  connections:
  Mechanical Translational Reference/LConn1 -- Ideal Force Sensor/RConn1
  Translational Friction/LConn1 -- Ideal Force Sensor/LConn1
  Translational Friction/RConn1 -- Ideal Translational Velocity Source/LConn1
  Ideal Force Sensor/RConn2 -- Joint Diameter/LConn1
  Joint Diameter/RConn1 -- Friction Torque/RConn1
  Mechanical Translational Reference1/LConn1 -- Ideal Translational Velocity Source/RConn2
  Joint Force/RConn1 -- PS Terminator/LConn1
  Joint Radius/LConn1 -- Joint Angular Velocity/RConn1
  Joint Radius/RConn1 -- Ideal Translational Velocity Source/RConn1

== system experiment_toplevel/GR Minitaur/minitaur_leg_linkages_IV/Joint Friction Model1/Stick-Slip ==
  Joint Diameter : fl_lib/Physical Signals/Functions/PS Gain  gain=2*leg_joint_radius
  Joint Radius : fl_lib/Physical Signals/Functions/PS Gain  gain=leg_joint_radius
  PS Add : fl_lib/Physical Signals/Functions/PS Add
  Stick-Slip Friction X : Contact_Forces_Lib/Friction Utilities/Stick-Slip Friction 1D  fn_axis=X-Axis  mu_kinetic=mu_k/2  mu_static=mu_s/2  vel_th=linear_region_thresh  filt_const=1/(2*pi*fric_bandwidth)
  Stick-Slip Friction Y : Contact_Forces_Lib/Friction Utilities/Stick-Slip Friction 1D  fn_axis=Y-Axis  mu_kinetic=mu_k/2  mu_static=mu_s/2  vel_th=linear_region_thresh  filt_const=1/(2*pi*fric_bandwidth)
  Joint Angular Velocity : PMIOPort  Port=1  Side=Left
  Joint Force : PMIOPort  Port=2  Side=Left
  Friction Torque : PMIOPort  Port=3  Side=Right
  connections:
  Joint Radius/RConn1 -- Stick-Slip Friction X/LConn2 -- Stick-Slip Friction Y/LConn2
  Joint Force/RConn1 -- Stick-Slip Friction X/LConn1 -- Stick-Slip Friction Y/LConn1
  Stick-Slip Friction Y/RConn1 -- PS Add/LConn2
  Stick-Slip Friction X/RConn1 -- PS Add/LConn1
  Joint Diameter/LConn1 -- PS Add/RConn1
  Joint Diameter/RConn1 -- Friction Torque/RConn1
  Joint Radius/LConn1 -- Joint Angular Velocity/RConn1

== system experiment_toplevel/GR Minitaur/minitaur_leg_linkages_IV/Joint Friction Model2/Full ==
  Ideal Force Sensor : fl_lib/Mechanical/Mechanical Sensors/Ideal Force Sensor
  Ideal Translational Velocity Source : fl_lib/Mechanical/Mechanical Sources/Ideal Translational Velocity Source
  Joint Diameter : fl_lib/Physical Signals/Functions/PS Gain  gain=2*leg_joint_radius
  Joint Radius : fl_lib/Physical Signals/Functions/PS Gain  gain=leg_joint_radius
  Mechanical Translational Reference : fl_lib/Mechanical/Translational Elements/Mechanical Translational Reference
  Mechanical Translational Reference1 : fl_lib/Mechanical/Translational Elements/Mechanical Translational Reference
  PS Terminator : fl_lib/Physical Signals/Sinks/PS Terminator
  Translational Friction : fl_lib/Mechanical/Translational Elements/Translational Friction  brkwy_frc=mu_brk*Fn N  Col_frc=mu_k*Fn N  visc_coef=fric_visc_coeff N/(m/s)  trans_coef=trans_coeff s/m  vel_thr=linear_region_thresh m/s  v_specify=off  v_priority=None  v=0 m/s  f_specify=off  f_priority=None  f=0 N
  Joint Angular Velocity : PMIOPort  Port=1  Side=Left
  Joint Force : PMIOPort  Port=2  Side=Left
  Friction Torque : PMIOPort  Port=3  Side=Right
  connections:
  Mechanical Translational Reference/LConn1 -- Ideal Force Sensor/RConn1
  Translational Friction/LConn1 -- Ideal Force Sensor/LConn1
  Translational Friction/RConn1 -- Ideal Translational Velocity Source/LConn1
  Ideal Force Sensor/RConn2 -- Joint Diameter/LConn1
  Joint Diameter/RConn1 -- Friction Torque/RConn1
  Mechanical Translational Reference1/LConn1 -- Ideal Translational Velocity Source/RConn2
  Joint Force/RConn1 -- PS Terminator/LConn1
  Joint Radius/LConn1 -- Joint Angular Velocity/RConn1
  Joint Radius/RConn1 -- Ideal Translational Velocity Source/RConn1

== system experiment_toplevel/GR Minitaur/minitaur_leg_linkages_IV/Joint Friction Model2/Stick-Slip ==
  Joint Diameter : fl_lib/Physical Signals/Functions/PS Gain  gain=2*leg_joint_radius
  Joint Radius : fl_lib/Physical Signals/Functions/PS Gain  gain=leg_joint_radius
  PS Add : fl_lib/Physical Signals/Functions/PS Add
  Stick-Slip Friction X : Contact_Forces_Lib/Friction Utilities/Stick-Slip Friction 1D  fn_axis=X-Axis  mu_kinetic=mu_k/2  mu_static=mu_s/2  vel_th=linear_region_thresh  filt_const=1/(2*pi*fric_bandwidth)
  Stick-Slip Friction Y : Contact_Forces_Lib/Friction Utilities/Stick-Slip Friction 1D  fn_axis=Y-Axis  mu_kinetic=mu_k/2  mu_static=mu_s/2  vel_th=linear_region_thresh  filt_const=1/(2*pi*fric_bandwidth)
  Joint Angular Velocity : PMIOPort  Port=1  Side=Left
  Joint Force : PMIOPort  Port=2  Side=Left
  Friction Torque : PMIOPort  Port=3  Side=Right
  connections:
  Joint Radius/RConn1 -- Stick-Slip Friction X/LConn2 -- Stick-Slip Friction Y/LConn2
  Joint Force/RConn1 -- Stick-Slip Friction X/LConn1 -- Stick-Slip Friction Y/LConn1
  Stick-Slip Friction Y/RConn1 -- PS Add/LConn2
  Stick-Slip Friction X/RConn1 -- PS Add/LConn1
  Joint Diameter/LConn1 -- PS Add/RConn1
  Joint Diameter/RConn1 -- Friction Torque/RConn1
  Joint Radius/LConn1 -- Joint Angular Velocity/RConn1

== system experiment_toplevel/GR Minitaur/minitaur_motor_module_IA/DYS_BLDC_86x10_BE8108_12/BLDC Model ==
  Desired Torque  [Nm] : Inport
  Velocity [rad/s] : Inport  Port=2
  Constant : Constant  Value=torque_sat
  Constant1 : Constant  Value=-torque_sat
  Gain : Gain  Gain=1/kt
  Gain1 : Gain  Gain=r
  Math Function : Math  Operator=square  SaturateOnIntegerOverflow=on
  Saturation Dynamic : simulink/Discontinuities/Saturation Dynamic  OutMin=[]  OutMax=[]  OutDataTypeStr=Inherit: Same as second input  OutDataType=fixdt(1, 16)  OutScaling=2^-10  DoSatur=off
  Terminator : Terminator
  Transfer Fcn : TransferFcn  Denominator=[timeconst 1]
  Torque [N*m] : Outport
  Ploss [W] : Outport  Port=2
  wires:
  Desired Torque  [Nm]/1 -> Transfer Fcn/1
  Math Function/1 -> Gain1/1
  Gain/1 -> Math Function/1
  Gain1/1 -> Ploss [W]/1
  Velocity [rad/s]/1 -> Terminator/1
  Transfer Fcn/1 -> Saturation Dynamic/2
  Saturation Dynamic/1 -> Gain/1, Torque [N*m]/1
  Constant/1 -> Saturation Dynamic/1
  Constant1/1 -> Saturation Dynamic/3

== system experiment_toplevel/GR Minitaur/minitaur_motor_module_IA/DYS_BLDC_86x10_BE8108_12/DYS_BLDC_86x10_BE8108_12_rotor_1_RIGID ==
  ReferenceFrame : sm_lib/Frames and Transforms/Reference Frame
  Solid : sm_lib/Body Elements/Solid  InertiaType=Custom  Mass=minitaurParams.Solid(7).mass  MassUnits=kg  CenterOfMass=minitaurParams.Solid(7).CoM  CenterOfMassUnits=mm  MomentsOfInertia=minitaurParams.Solid(7).MoI  MomentsOfInertiaUnits=kg*mm^2  ProductsOfInertia=minitaurParams.Solid(7).PoI  ProductsOfInertiaUnits=kg*mm^2  DensityBased=on  Density=1000  DensityUnits=kg/(m^3)  DoExposeReferenceFrame=on  SerializedFrames=<Frames/>  GraphicType=FromGeometry  MarkerShape=Sphere  MarkerSize=10  GraphicVisPropType=SimpleVisualProperties  GraphicDiffuseColor=minitaurParams.Solid(7).color  GraphicSpecularColor=[0.5 0.5 0.5 1.0]  GraphicAmbientColor=[0.15 0.15 0.15 1.0]  GraphicEmissiveColor=[0.0 0.0 0.0 1.0]  GraphicShininess=75  GraphicOpacity=minitaurParams.Solid(7).opacity  GeometryShape=FromFile  RectangleSize=[1 1]  RectangleSizeUnits=m  BrickDimensions=[1 1 1]  BrickDimensionUnits=m  CylinderRadius=1  CylinderRadiusUnits=m  CylinderLength=1  CylinderLengthUnits=m  SphereRadius=1  SphereRadiusUnits=m  EllipsoidRadii=[1 1 1]  EllipsoidRadiiUnits=m  ExtrusionCrossSection=[1 1; -1 1; -1 -1; 1 -1]  ExtrusionCrossSectionUnits=m  ExtrusionLength=1  ExtrusionLengthUnits=m  PolygonNumSides=3  PolygonOuterRadius=1  PolygonOuterRadiusUnits=m  ExtGeomFileType=STEP  ExtGeomFileName=model/DYS-BLDC-86x10-BE8108-12-rotor_Default_sldprt.STEP  ExtGeomFileUnits=m  RevolutionCrossSection=[1 1; 1 -1; 2 -1; 2 1]  RevolutionCrossSectionUnits=m  RevolutionExtent=Full  RevolutionAngle=180  RevolutionAngleUnits=deg
  Transform : sm_lib/Frames and Transforms/Rigid Transform  TranslationMethod=Cartesian  TranslationLengthUnit=mm  TranslationStandardAxis=+Z  TranslationStandardOffset=0  TranslationCartesianOffset=minitaurParams.RigidTransform(20).translation  TranslationROffset=0  TranslationROffsetUnits=m  TranslationZOffset=0  TranslationZOffsetUnits=m  TranslationThetaOffset=0  TranslationThetaOffsetUnits=deg  RotationMethod=ArbitraryAxis  RotationAngleUnits=rad  RotationStandardAxis=+Z  RotationAngle=minitaurParams.RigidTransform(20).angle  RotationArbitraryAxis=minitaurParams.RigidTransform(20).axis  FollAlignAxisA=+X  BaseAlignAxisA=+Y  FollAlignAxisB=+Y  BaseAlignAxisB=+Z  RotationSequenceAxes=FollowerAxes  RotationSequence=XYX  RotationSequenceAngles=[0 0 0]  RotationSequenceAnglesUnits=deg  RotationMatrix=[1 0 0; 0 1 0; 0 0 1]
  Transform1 : sm_lib/Frames and Transforms/Rigid Transform  TranslationMethod=Cartesian  TranslationLengthUnit=mm  TranslationStandardAxis=+Z  TranslationStandardOffset=0  TranslationCartesianOffset=minitaurParams.RigidTransform(48).translation  TranslationROffset=0  TranslationROffsetUnits=m  TranslationZOffset=0  TranslationZOffsetUnits=m  TranslationThetaOffset=0  TranslationThetaOffsetUnits=deg  RotationMethod=ArbitraryAxis  RotationAngleUnits=rad  RotationStandardAxis=+Z  RotationAngle=minitaurParams.RigidTransform(48).angle  RotationArbitraryAxis=minitaurParams.RigidTransform(48).axis  FollAlignAxisA=+X  BaseAlignAxisA=+Y  FollAlignAxisB=+Y  BaseAlignAxisB=+Z  RotationSequenceAxes=FollowerAxes  RotationSequence=XYX  RotationSequenceAngles=[0 0 0]  RotationSequenceAnglesUnits=deg  RotationMatrix=[1 0 0; 0 1 0; 0 0 1]
  F1 : PMIOPort  Port=1  Side=Left
  F : PMIOPort  Port=2  Side=Left
  connections:
  ReferenceFrame/RConn1 -- Solid/RConn1 -- Transform/LConn1 -- Transform1/LConn1
  Transform/RConn1 -- F/RConn1
  Transform1/RConn1 -- F1/RConn1
